simulink model "NECK_TRUTH_ASSEMBLY"  (R2021b)
settings: Solver=daessc  StartTime=0.0  StopTime=11  MaxStep=1e-3  RelTol=1e-3
model workspace (MAT data in the model file):
  Ts = 0.001
  smiData.RigidTransform(1).translation = [0 44.1311004689 0]
  smiData.RigidTransform(1).angle = 2.09439510239
  smiData.RigidTransform(1).axis = [0.57735026919 -0.57735026919 0.57735026919]
  smiData.RigidTransform(1).ID = 'B[61:-:64]'
  smiData.RigidTransform(2).translation = [44.1311004689 0 0]
  smiData.RigidTransform(2).angle = 2.09439510239
  smiData.RigidTransform(2).axis = [-0.57735026919 -0.57735026919 0.57735026919]
  smiData.RigidTransform(2).ID = 'F[61:-:64]'
  smiData.RigidTransform(3).translation = [2.38869129525e-15 -9.5 -21.05]
  smiData.RigidTransform(3).angle = 1.22460635382e-16
  smiData.RigidTransform(3).axis = [0 1 0]
  smiData.RigidTransform(3).ID = 'B[64:-:65]'
  smiData.RigidTransform(4).translation = [3.5527136788e-15 -9.5 -21.05]
  smiData.RigidTransform(4).angle = 2.8305244335e-16
  smiData.RigidTransform(4).axis = [0.196116135138 0.980580675691 2.72165810914e-17]
  smiData.RigidTransform(4).ID = 'F[64:-:65]'
  smiData.RigidTransform(5).translation = [0 0 0]
  smiData.RigidTransform(5).angle = 0
  smiData.RigidTransform(5).axis = [0 0 0]
  smiData.RigidTransform(5).ID = 'B[65:-:66]'
  smiData.RigidTransform(6).translation = [-6.31088724177e-30 -2.10384225914e-15 1.45125838727e-14]
  smiData.RigidTransform(6).angle = 0
  smiData.RigidTransform(6).axis = [0 0 0]
  smiData.RigidTransform(6).ID = 'F[65:-:66]'
  smiData.RigidTransform(7).translation = [0 0 0]
  smiData.RigidTransform(7).angle = 0
  smiData.RigidTransform(7).axis = [0 0 0]
  smiData.RigidTransform(7).ID = 'B[66:-:69]'
  smiData.RigidTransform(8).translation = [-2.73406886406e-15 -1.42108547152e-14 2.50841014626e-14]
  smiData.RigidTransform(8).angle = 0
  smiData.RigidTransform(8).axis = [0 0 0]
  smiData.RigidTransform(8).ID = 'F[66:-:69]'
  smiData.RigidTransform(9).translation = [0 0 0]
  smiData.RigidTransform(9).angle = 0
  smiData.RigidTransform(9).axis = [0 0 0]
  smiData.RigidTransform(9).ID = 'SixDofRigidTransform[61]'
  smiData.Solid(1).mass = 0
  smiData.Solid(1).CoM = [0 0 0]
  smiData.Solid(1).MoI = [0 0 0]
  smiData.Solid(1).PoI = [0 0 0]
  smiData.Solid(1).color = [0 0.6 0.8]
  smiData.Solid(1).opacity = 1
  smiData.Solid(1).ID = 'NECK_TRUTH_SKEL_prt'
  smiData.Solid(2).mass = 0.125390378189
  smiData.Solid(2).CoM = [-0.0363551448448 -6.61926182163 -6.38188077777]
  smiData.Solid(2).MoI = [40.5180614905 38.6502416268 47.3631511196]
  smiData.Solid(2).PoI = [-9.37947339067 0.0999862574752 0.0590587986716]
  smiData.Solid(2).color = [0.5 0.5 0.5]
  smiData.Solid(2).opacity = 1
  smiData.Solid(2).ID = 'SIM_HEAD_NECK_2_PITCH_prt'
  smiData.Solid(3).mass = 0.189999387789
  smiData.Solid(3).CoM = [0.0824235199086 -45.5984632245 1.26608008716]
  smiData.Solid(3).MoI = [123.735798883 41.2768779908 110.667550367]
  smiData.Solid(3).PoI = [-10.3140357148 -0.372253294164 -0.541348054696]
  smiData.Solid(3).color = [0.5 0.5 0.5]
  smiData.Solid(3).opacity = 1
  smiData.Solid(3).ID = 'SIM_HEAD_NECK_3_ROLL_prt'
  smiData.Solid(4).mass = 0.0295418901539
  smiData.Solid(4).CoM = [-0.000680150826415 -69.2520020375 0.535664257451]
  smiData.Solid(4).MoI = [2.57045773244 2.07153450679 2.53671405207]
  smiData.Solid(4).PoI = [0.161333413847 0 0.000259130776769]
  smiData.Solid(4).color = [0.5 0.5 0.5]
  smiData.Solid(4).opacity = 1
  smiData.Solid(4).ID = 'SIM_HEAD_NECK_4_YAW_prt'
  smiData.Solid(5).mass = 1.91786952499
  smiData.Solid(5).CoM = [0.012492365855 -107.103598511 -14.802582146]
  smiData.Solid(5).MoI = [11921.8024422 12787.4091291 10368.3301757]
  smiData.Solid(5).PoI = [-35.4825090084 0.17432139015 -0.295251965821]
  smiData.Solid(5).color = [0.5 0.5 0.5]
  smiData.Solid(5).opacity = 1
  smiData.Solid(5).ID = 'SIM_HEAD_HEAD_2_prt'
  smiData.RevoluteJoint(1).Rz.Pos = 0
  smiData.RevoluteJoint(1).ID = '[61:-:64]'
  smiData.RevoluteJoint(2).Rz.Pos = -2.86249921332e-14
  smiData.RevoluteJoint(2).ID = '[64:-:65]'
libraries: slpidlib x2, robotcorelib x1, simulink x1
settings Model: Creator=mfussi  LastModifiedBy=mfussi
settings ExplorerConfigSet: InternalSimMechanicsExplorerSettings="<ExplorerConfiguration><canonicalview>default</canonicalview><AnimationSetting><BasePlaybackSpeed>1.0</BasePlaybackSpeed><PlaybackSpeedFactor>1.0</PlaybackSpeedFactor></AnimationSetting><TilePanel><TileInfo><Tiles Columns=\"2\" Count=\"3\" Rows=\"2\"><Column Weight=\"0.463\"/><Column Weight=\"0.537\"/><Row Weight=\"0.4995\"/><Row Weight=\"0.5005\"/><Tile Height=\"2\" Width=\"1\" X=\"0\" Y=\"0\"/><Tile Height=\"1\" Width=\"1\" X=\"1\" Y=\"0\"/><Tile Height=\"1\" Width=\"1\" X=\"1\" Y=\"1\"/></Tiles></TileInfo><SceneInfo><SceneViewer><BGColor><R>1</R><G>1</G><B>1</B></BGColor><Camera><DoPerspective>off</DoPerspective><Position><X>0.560529878452456387</X><Y>-0.579308542829303552</Y><Z>0.688271017729185863</Z></Position><Center><X>-0.0168203907371694134</X><Y>-0.00195827363967777512</Y><Z>0.110920748539560035</Z></Center><Up><X>-0.408248290463863073</X><Y>0.408248290463863073</Y><Z>0.816496580927726145</Z></Up><ViewLimDist>1</ViewLimDist><YLim>0.202462271511554742</YLim><XLim>0.155950668596738118</XLim></Camera></SceneViewer><SceneViewer><BGColor><R>1</R><G>1</G><B>1</B></BGColor><Camera><DoPerspective>off</DoPerspective><Position><X>-0.00907661192889466263</X><Y>-1.00002945628579276</Y><Z>0.0987252115554740212</Z></Position><Center><X>-0.00907661192889466263</X><Y>-2.94562857927754829e-05</Y><Z>0.0987252115554740212</Z></Center><Up><X>0</X><Y>-0</Y><Z>1</Z></Up><ViewLimDist>1</ViewLimDist><YLim>0.125749995959142186</YLim><XLim>0.226742195442897698</XLim></Camera></SceneViewer><SceneViewer><BGColor><R>1</R><G>1</G><B>1</B></BGColor><Camera><DoPerspective>off</DoPerspective><Position><X>0.983678532336833777</X><Y>-0.000360963789647767157</Y><Z>0.0904901561375027336</Z></Position><Center><X>-0.0163214676631662226</X><Y>-0.000360963789647767157</Y><Z>0.0904901561375027336</Z></Center><Up><X>-0</X><Y>0</Y><Z>1</Z></Up><ViewLimDist>1</ViewLimDist><YLim>0.121003071725368519</YLim><XLim>0.217758446198377198</XLim></Camera></SceneViewer></SceneInfo></TilePanel><MechEditorPanel><Cameras/><GfxPanelCameraMap/><VideoCreator><PlaybackSpeedRatio>1.0</PlaybackSpeedRatio><FrameRate>30</FrameRate><VideoFormat>MPEG-4</VideoFormat><FrameSize>[1280 720]</FrameSize></VideoCreator></MechEditorPanel></ExplorerConfiguration>"

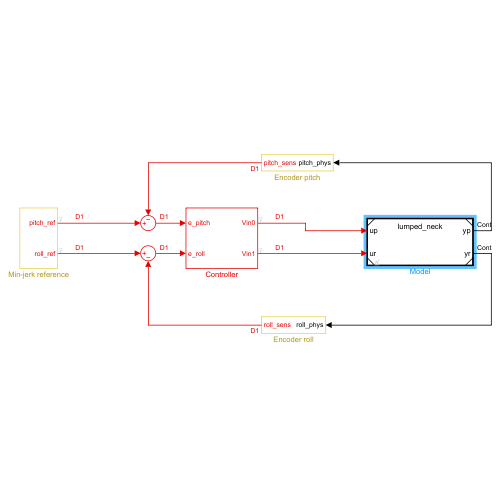
[thumbnail: Simulink's stored preview of the top-level diagram]
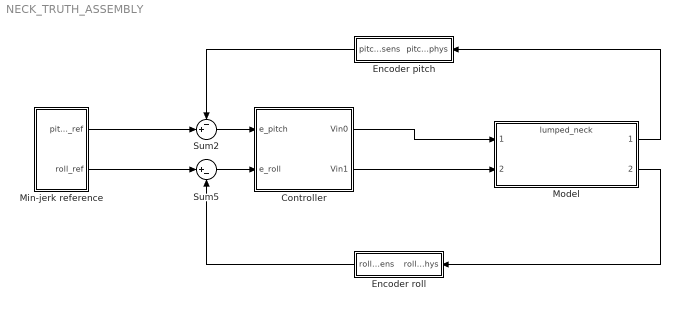
== system NECK_TRUTH_ASSEMBLY ==
  Controller : Subsystem
  Encoder pitch : Subsystem
  Encoder roll : Subsystem
  Min-jerk reference : Subsystem
  Model : ModelReference  ModelNameDialog=lumped_neck.slx  SimulationMode=Normal  ModelReferenceVersion=1.6
  Sum2 : Sum  Inputs=-+|
  Sum5 : Sum  Inputs=|+-
  wires:
  Min-jerk reference/1(pitch_ref) -> Sum2/2
  Min-jerk reference/2(roll_ref) -> Sum5/1
  Encoder pitch/1(pitch_sens) -> Sum2/1
  Encoder roll/1(roll_sens) -> Sum5/2
  Sum2/1 -> Controller/1(e_pitch)
  Sum5/1 -> Controller/2(e_roll)
  Controller/2(Vin1) -> Model/2
  Controller/1(Vin0) -> Model/1
  Model/2 -> Encoder roll/1(roll_phys)
  Model/1 -> Encoder pitch/1(pitch_phys)

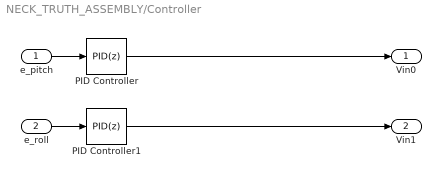
== system NECK_TRUTH_ASSEMBLY/Controller ==
  e_pitch : Inport
  e_roll : Inport  Port=2
  PID Controller : slpidlib/PID Controller  Controller=PID  Form=Parallel  TimeDomain=Discrete-time  UseExternalTs=off  SampleTime=Ts  IntegratorMethod=Trapezoidal  FilterMethod=Forward Euler  ControllerParametersSource=internal  P=3.23300595070019  I=22.7597079107816  D=0.108833361497331  UseFilter=on  N=662.901994136113  TunerSelectOption=Transfer Function Based (PID Tuner App)  InitialConditionSource=internal  InitialConditionForIntegrator=0  InitialConditionForFilter=0  DifferentiatorICPrevScaledInput=0  ExternalReset=none  TrackingMode=off  Kt=1  LimitOutput=off  SatLimitsSource=internal  UpperSaturationLimit=inf  LowerSaturationLimit=-inf  LinearizeAsGain=on  AntiWindupMode=none  Kb=1  POutMin=[]  POutMax=[]  IOutMin=[]  IOutMax=[]  DOutMin=[]  DOutMax=[]  NOutMin=[]  NOutMax=[]  SumOutMin=[]  SumOutMax=[]  SaturationOutMin=[]  SaturationOutMax=[]  PParamMin=[]  PParamMax=[]  IParamMin=[]  IParamMax=[]  DParamMin=[]  DParamMax=[]  NParamMin=[]  NParamMax=[]  KbParamMin=[]  KbParamMax=[]  KtParamMin=[]  KtParamMax=[]  KbOutMin=[]  KbOutMax=[]  KtOutMin=[]  KtOutMax=[]  IntegratorOutMin=[]  IntegratorOutMax=[]  FilterOutMin=[]  FilterOutMax=[]  SumI1OutMin=[]  SumI1OutMax=[]  SumI2OutMin=[]  SumI2OutMax=[]  SumI3OutMin=[]  SumI3OutMax=[]  SumI4OutMin=[]  SumI4OutMax=[]  SumDOutMin=[]  SumDOutMax=[]  DifferentiatorOutMin=[]  DifferentiatorOutMax=[]  FilterDiffOutCoefMin=[]  FilterDiffOutCoefMax=[]  ReciprocalOutMin=[]  ReciprocalOutMax=[]  SumDenOutMin=[]  SumDenOutMax=[]  SumNumOutMin=[]  SumNumOutMax=[]  DivideOutMin=[]  DivideOutMax=[]  UdiffTsProdOutMin=[]  UdiffTsProdOutMax=[]  NTsProdOutMin=[]  NTsProdOutMax=[]  UintegralTsProdOutMin=[]  UintegralTsProdOutMax=[]  UngainTsProdOutMin=[]  UngainTsProdOutMax=[]  IntegratorContinuousStateAttributes=''  IntegratorStateMustResolveToSignalObject=off  IntegratorRTWStateStorageClass=Auto  FilterContinuousStateAttributes=''  FilterStateMustResolveToSignalObject=off  FilterRTWStateStorageClass=Auto  ParallelPVariant=InternalParameters  IdealPVariant=Disabled  IVariant=InternalParameters  DVariant=InternalParameters  IntegratorVariant=Discrete  SatVariant=Disabled  AWVariant=Passthrough  PCopyVariant=Disabled  TRVariant=Disabled  FdbkBlocksVariant=Forward  IdealPFdbkVariant=Disabled  SatFdbkVariant=Disabled  DerivativeFilterVariant=ForwardEulerFilter  NVariant=InternalParameters  NCopyVariant=Disabled  FilterICVariant=InternalICsFilter  IntegratorICVariant=InternalICs  ExternalResetVariant=Disabled  TRSumVariant=Passthrough  SumFdbkVariant=Disabled  SumVariant=Sum_PID  TsampFilterVariant=InternalTs  TsampNgainVariant=Passthrough  TsampIntegralVariant=Passthrough  ExternalSaturationOutDataTypeStr=Inherit: Same as second input
  PID Controller1 : slpidlib/PID Controller  Controller=PID  Form=Parallel  TimeDomain=Discrete-time  UseExternalTs=off  SampleTime=Ts  IntegratorMethod=Trapezoidal  FilterMethod=Forward Euler  ControllerParametersSource=internal  P=1.0021029432336  I=2.65241768173488  D=0.048221588844032  UseFilter=on  N=1692.09219805413  TunerSelectOption=Transfer Function Based (PID Tuner App)  InitialConditionSource=internal  InitialConditionForIntegrator=0  InitialConditionForFilter=0  DifferentiatorICPrevScaledInput=0  ExternalReset=none  TrackingMode=off  Kt=1  LimitOutput=off  SatLimitsSource=internal  UpperSaturationLimit=inf  LowerSaturationLimit=-inf  LinearizeAsGain=on  AntiWindupMode=none  Kb=1  POutMin=[]  POutMax=[]  IOutMin=[]  IOutMax=[]  DOutMin=[]  DOutMax=[]  NOutMin=[]  NOutMax=[]  SumOutMin=[]  SumOutMax=[]  SaturationOutMin=[]  SaturationOutMax=[]  PParamMin=[]  PParamMax=[]  IParamMin=[]  IParamMax=[]  DParamMin=[]  DParamMax=[]  NParamMin=[]  NParamMax=[]  KbParamMin=[]  KbParamMax=[]  KtParamMin=[]  KtParamMax=[]  KbOutMin=[]  KbOutMax=[]  KtOutMin=[]  KtOutMax=[]  IntegratorOutMin=[]  IntegratorOutMax=[]  FilterOutMin=[]  FilterOutMax=[]  SumI1OutMin=[]  SumI1OutMax=[]  SumI2OutMin=[]  SumI2OutMax=[]  SumI3OutMin=[]  SumI3OutMax=[]  SumI4OutMin=[]  SumI4OutMax=[]  SumDOutMin=[]  SumDOutMax=[]  DifferentiatorOutMin=[]  DifferentiatorOutMax=[]  FilterDiffOutCoefMin=[]  FilterDiffOutCoefMax=[]  ReciprocalOutMin=[]  ReciprocalOutMax=[]  SumDenOutMin=[]  SumDenOutMax=[]  SumNumOutMin=[]  SumNumOutMax=[]  DivideOutMin=[]  DivideOutMax=[]  UdiffTsProdOutMin=[]  UdiffTsProdOutMax=[]  NTsProdOutMin=[]  NTsProdOutMax=[]  UintegralTsProdOutMin=[]  UintegralTsProdOutMax=[]  UngainTsProdOutMin=[]  UngainTsProdOutMax=[]  IntegratorContinuousStateAttributes=''  IntegratorStateMustResolveToSignalObject=off  IntegratorRTWStateStorageClass=Auto  FilterContinuousStateAttributes=''  FilterStateMustResolveToSignalObject=off  FilterRTWStateStorageClass=Auto  ParallelPVariant=InternalParameters  IdealPVariant=Disabled  IVariant=InternalParameters  DVariant=InternalParameters  IntegratorVariant=Discrete  SatVariant=Disabled  AWVariant=Passthrough  PCopyVariant=Disabled  TRVariant=Disabled  FdbkBlocksVariant=Forward  IdealPFdbkVariant=Disabled  SatFdbkVariant=Disabled  DerivativeFilterVariant=ForwardEulerFilter  NVariant=InternalParameters  NCopyVariant=Disabled  FilterICVariant=InternalICsFilter  IntegratorICVariant=InternalICs  ExternalResetVariant=Disabled  TRSumVariant=Passthrough  SumFdbkVariant=Disabled  SumVariant=Sum_PID  TsampFilterVariant=InternalTs  TsampNgainVariant=Passthrough  TsampIntegralVariant=Passthrough  ExternalSaturationOutDataTypeStr=Inherit: Same as second input
  Vin0 : Outport
  Vin1 : Outport  Port=2
  wires:
  e_roll/1 -> PID Controller1/1
  PID Controller/1 -> Vin0/1
  e_pitch/1 -> PID Controller/1
  PID Controller1/1 -> Vin1/1

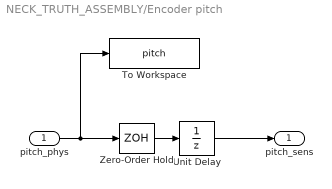
== system NECK_TRUTH_ASSEMBLY/Encoder pitch ==
  pitch_phys : Inport
  To Workspace : ToWorkspace  VariableName=pitch  SaveFormat=Timeseries  SampleTime=-1
  Unit Delay : UnitDelay  SampleTime=Ts  HasFrameUpgradeWarning=on
  Zero-Order Hold : ZeroOrderHold  SampleTime=Ts
  pitch_sens : Outport
  wires:
  Unit Delay/1 -> pitch_sens/1
  pitch_phys/1 -> Zero-Order Hold/1, To Workspace/1
  Zero-Order Hold/1 -> Unit Delay/1

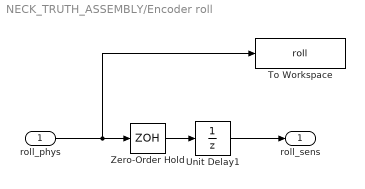
== system NECK_TRUTH_ASSEMBLY/Encoder roll ==
  roll_phys : Inport
  To Workspace : ToWorkspace  VariableName=roll  SaveFormat=Timeseries  SampleTime=-1
  Unit Delay1 : UnitDelay  SampleTime=Ts  HasFrameUpgradeWarning=on
  Zero-Order Hold : ZeroOrderHold  SampleTime=Ts
  roll_sens : Outport
  wires:
  Unit Delay1/1 -> roll_sens/1
  roll_phys/1 -> Zero-Order Hold/1, To Workspace/1
  Zero-Order Hold/1 -> Unit Delay1/1

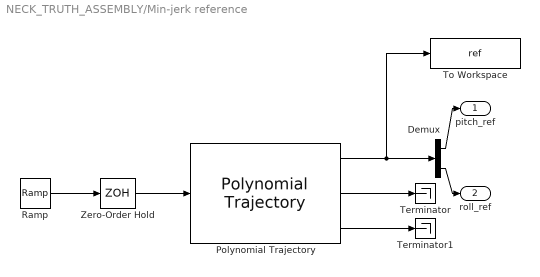
== system NECK_TRUTH_ASSEMBLY/Min-jerk reference ==
  Demux : Demux  Outputs=2
  Polynomial Trajectory : robotcorelib/Polynomial Trajectory  WaypointSource=Internal  Waypoints=wp  TimePoints=tp  TimeInterval=[ 1, 4 ]  Method=Quintic Polynomial  ParameterSource=Internal  VelocityBoundaryCondition=vel_bounds  AccelerationBoundaryCondition=accel_bounds  SimulateUsing=Code generation
  Ramp : simulink/Sources/Ramp  slope=1  start=0  InitialOutput=0
  Terminator : Terminator
  Terminator1 : Terminator
  To Workspace : ToWorkspace  VariableName=ref  SaveFormat=Timeseries  SampleTime=-1
  Zero-Order Hold : ZeroOrderHold  SampleTime=-1
  pitch_ref : Outport
  roll_ref : Outport  Port=2
  wires:
  Polynomial Trajectory/3 -> Terminator1/1
  Polynomial Trajectory/1 -> To Workspace/1, Demux/1
  Polynomial Trajectory/2 -> Terminator/1
  Ramp/1 -> Zero-Order Hold/1
  Demux/1 -> pitch_ref/1
  Zero-Order Hold/1 -> Polynomial Trajectory/1
  Demux/2 -> roll_ref/1
